simulink library "Meldas_library"  (R2018a)
settings: Solver=VariableStepAuto  StartTime=0.0  StopTime=10.0  RelTol=1e-3
undefined symbols (not defined in the file or in its folder): Cf, Iz, lf, m
settings Model: Creator=mulusoy  LastModifiedBy=mulusoy

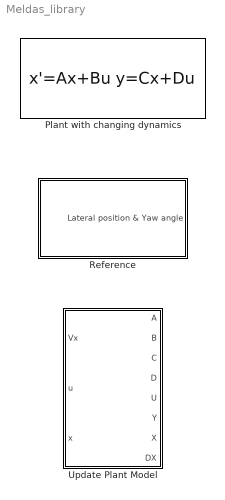
== system Meldas_library ==
  Plant with changing dynamics : StateSpace  A=|  B=[2*Cf/m 0 2*Cf*lf/Iz 0]';  C=[0 0 0 1; 0 1 0 0];  D=[0;0]  InitialCondition=0  mask{Vx=15}
      | [-(2*Cf+2*Cr)/m/Vx, 0, -Vx-(2*Cf*lf-2*Cr*lr)/m/Vx, 0;
      |      0, 0, 1, 0;
      |      -(2*Cf*lf-2*Cr*lr)/Iz/Vx, 0, -(2*Cf*lf^2+2*Cr*lr^2)/Iz/Vx, 0;
      |      1, Vx, 0, 0];
      mask Display: image("car.jpg")
  Reference : Subsystem
      mask Display: image("mask.jpg");
  Update Plant Model : MATLAB Function  TreatAsAtomicUnit=on

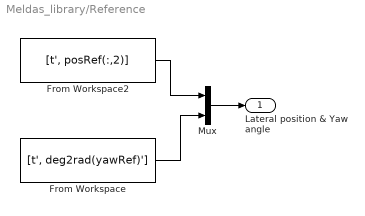
== system Meldas_library/Reference ==
  From Workspace : FromWorkspace  VariableName=[t', deg2rad(yawRef)']  SampleTime=0.1
  From Workspace2 : FromWorkspace  VariableName=[t', posRef(:,2)]  SampleTime=0.1
  Mux : Mux  Inputs=2
  Lateral position & Yaw angle : Outport
  wires:
  Mux/1 -> Lateral position & Yaw angle/1
  From Workspace/1 -> Mux/2
  From Workspace2/1 -> Mux/1

== matlab function Meldas_library/Update Plant Model ==
  data: Vx input; u input; A output size=[4,4]; x input size=[4,1]; B output size=[4,1]; C output size=[2,4]; D output size=[2,1]; U output; Y output size=[2,1]; X output size=[4,1]; DX output size=[4,1]
function [A,B,C,D,U,Y,X,DX] = fcn(Vx,u,x)
% Sample time
Ts = 0.1;

% Model parameters
m = 1575;
Iz = 2875;
lf = 1.2;
lr = 1.6;
Cf = 19000;
Cr = 33000;

% Continuous-time model
Ac = [-(2*Cf+2*Cr)/m/Vx, 0, -Vx-(2*Cf*lf-2*Cr*lr)/m/Vx, 0;
     0, 0, 1, 0;
     -(2*Cf*lf-2*Cr*lr)/Iz/Vx, 0, -(2*Cf*lf^2+2*Cr*lr^2)/Iz/Vx, 0;
     1, Vx, 0, 0];
Bc = [2*Cf/m 0 2*Cf*lf/Iz 0]';   
Cc = [0 0 0 1; 0 1 0 0];
Dc = zeros(2,1);

% Discretize the continuous-time model using zero-order hold 
% on the inputs and a sample time of Ts seconds
nx = size(Ac,1);
nu = size(Bc,2);
M = expm([[Ac Bc]*Ts; zeros(nu,nx+nu)]);
A = M(1:nx,1:nx);
B = M(1:nx,nx+1:nx+nu);
C = Cc;
D = Dc;

% Nominal conditions for discrete-time plant
X = x;
U = u;
Y = C*x + D*u;
DX = A*x+B*u-x;
